simulink subsystem "Elevator_sub"  (R2023b)
settings: Solver=VariableStepAuto  StartTime=0.0  StopTime=10.0  RelTol=1e-3
undefined symbols (not defined in the file): Elevator_Height_L1, Elevator_Height_L2, Elevator_Height_L3, Elevator_Height_L4, Elevator_Height_Pickup
libraries: simulink x5, Controls_Components_lib x1
settings Model: Creator=ander  LastModifiedBy=ander

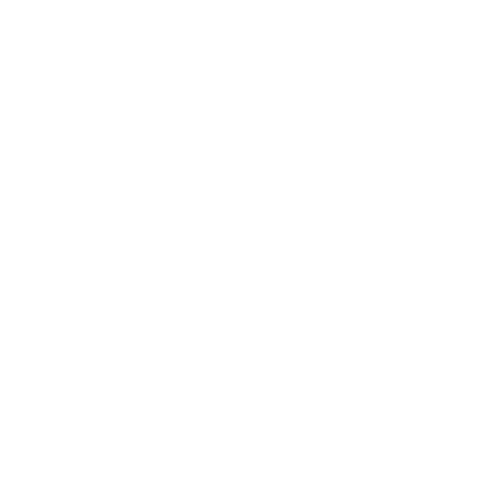
[thumbnail: Simulink's stored preview of the top-level diagram]
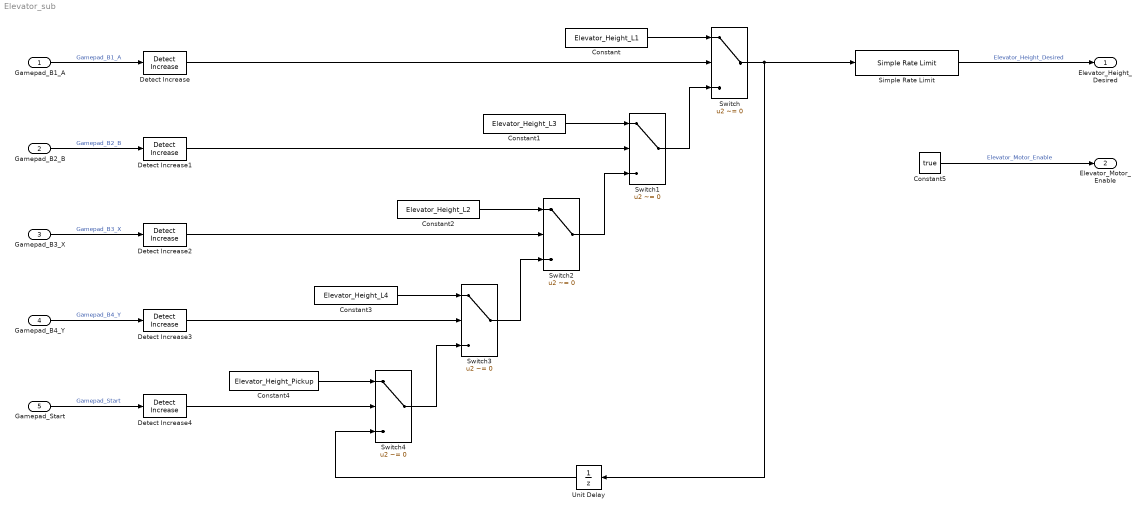
== system Elevator_sub ==
  Gamepad_B1_A : Inport
  Gamepad_B2_B : Inport  Port=2
  Gamepad_B3_X : Inport  Port=3
  Gamepad_B4_Y : Inport  Port=4
  Gamepad_Start : Inport  Port=5
  Constant : Constant  Value=Elevator_Height_L1
  Constant1 : Constant  Value=Elevator_Height_L3
  Constant2 : Constant  Value=Elevator_Height_L2
  Constant3 : Constant  Value=Elevator_Height_L4
  Constant4 : Constant  Value=Elevator_Height_Pickup
  Constant5 : Constant  Value=true
  Detect Increase{,1..4} (5 alike) : simulink/Logic and Bit Operations/Detect Increase  vinit=0.0  OutDataTypeStr=boolean
  Simple Rate Limit : Controls_Components_lib/Simple Rate Limit  Rate_Limit_Inc=Elevator_Height_RL_Inc  Rate_Limit_Dec=Elevator_Height_RL_Dec
  Switch{,1..4} (5 alike) : Switch  Criteria=u2 ~= 0  SaturateOnIntegerOverflow=off  InputSameDT=off
  Unit Delay : UnitDelay  SampleTime=-1  HasFrameUpgradeWarning=on
  Elevator_Height_Desired : Outport
  Elevator_Motor_Enable : Outport  Port=2
  wires:
  Gamepad_B1_A/1 -> Detect Increase/1  "Gamepad_B1_A"
  Gamepad_B2_B/1 -> Detect Increase1/1  "Gamepad_B2_B"
  Gamepad_B3_X/1 -> Detect Increase2/1  "Gamepad_B3_X"
  Gamepad_B4_Y/1 -> Detect Increase3/1  "Gamepad_B4_Y"
  Gamepad_Start/1 -> Detect Increase4/1  "Gamepad_Start"
  Detect Increase/1 -> Switch/2
  Constant/1 -> Switch/1
  Constant1/1 -> Switch1/1
  Detect Increase1/1 -> Switch1/2
  Detect Increase2/1 -> Switch2/2
  Constant2/1 -> Switch2/1
  Constant3/1 -> Switch3/1
  Detect Increase3/1 -> Switch3/2
  Detect Increase4/1 -> Switch4/2
  Constant4/1 -> Switch4/1
  Switch4/1 -> Switch3/3
  Switch3/1 -> Switch2/3
  Switch2/1 -> Switch1/3
  Switch1/1 -> Switch/3
  Switch/1 -> Unit Delay/1, Simple Rate Limit/1
  Unit Delay/1 -> Switch4/3
  Constant5/1 -> Elevator_Motor_Enable/1  "Elevator_Motor_Enable"
  Simple Rate Limit/1 -> Elevator_Height_Desired/1  "Elevator_Height_Desired"
